simulink model "Problem1"  (R2020b)
settings: Solver=VariableStepAuto  StartTime=0.0  StopTime=100  RelTol=1e-3
settings Model: Creator=omkar  LastModifiedBy=omkar

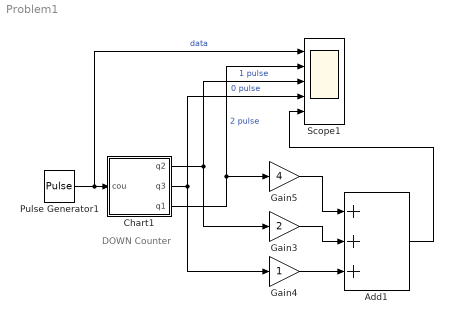
== system Problem1 ==
  note: DOWN Counter
  Add1 : Sum  Inputs=+++
  Chart1 : Stateflow chart  TreatAsAtomicUnit=on
  Gain3 : Gain  Gain=2
  Gain4 : Gain
  Gain5 : Gain  Gain=4
  Pulse Generator1 : DiscretePulseGenerator  PulseType=Time based  Period=10  PulseWidth=50
  Scope1 : Scope  NumInputPorts=5
  wires:
  Gain3/1 -> Add1/2
  Gain5/1 -> Add1/1
  Chart1/3(q1) -> Gain5/1, Scope1/2  "2 pulse"
  Chart1/2(q3) -> Gain4/1, Scope1/4  "0 pulse"
  Chart1/1(q2) -> Scope1/3, Gain3/1  "1 pulse"
  Add1/1 -> Scope1/5
  Pulse Generator1/1 -> Scope1/1, Chart1/1(cou)  "data"
  Gain4/1 -> Add1/3

== stateflow chart Problem1/Chart1 ==
  state a_case5
    entry:
    q1=1;
    q2=0;
    q3=0;
  state a_case1
    entry:
    q1=0;
    q2=0;
    q3=0;
  state a000
    entry:
    q1=0;
    q2=0;
    q3=0;
  state a0004
    entry:
    q1=1;
    q2=0;
    q3=0;
  state a0001
    entry:
    q1=0;
    q2=0;
    q3=1;
  state a_case4
    entry:
    q1=0;
    q2=1;
    q3=1;
  state a_case2
    entry:
    q1=0;
    q2=0;
    q3=1;
  state a0003
    entry:
    q1=0;
    q2=1;
    q3=1;
  state a0002
    entry:
    q1=0;
    q2=1;
    q3=0;
  state a_case3
    entry:
    q1=0;
    q2=1;
    q3=0;
  (default) -> a000
  a000 -> a_case5 : [cou==1]
  a_case1 -> a000 : [cou==0]
  a_case5 -> a0004 : [cou==0]
  a0001 -> a_case1 : [cou==1]
  a0004 -> a_case4 : [cou==1]
  a_case2 -> a0001 : [cou==0]
  a_case4 -> a0003 : [cou==0]
  a0002 -> a_case2 : [cou==1]
  a0003 -> a_case3 : [cou==1]
  a_case3 -> a0002 : [cou==0]
  data: q2 output; q3 output; q1 output; cou input
